simulink model "Navigation"  (R2021b)
settings: Solver=VariableStepAuto  StartTime=0.0  StopTime=10.0  RelTol=1e-3
settings Model: Creator=camil  LastModifiedBy=Paul

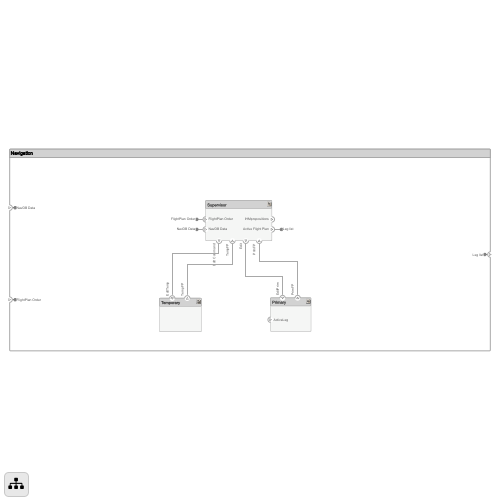
[thumbnail: Simulink's stored preview of the top-level diagram]
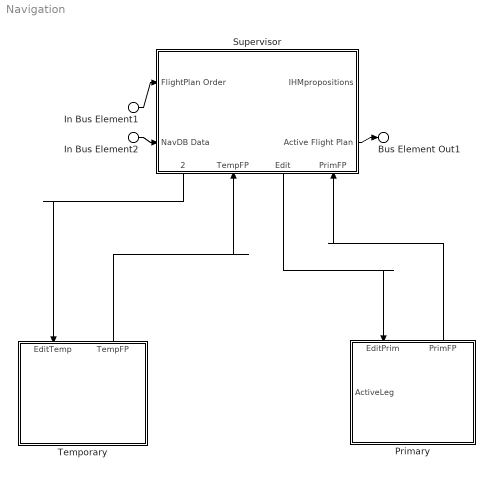
== system Navigation ==
  In Bus Element2 : Inport  PortName=NavDB Data
  In Bus Element1 : Inport  Port=2  PortName=FlightPlan Order
  Primary : Subsystem
      settings: PortSchema="{\"entries\":[{\"content\":{\"headerSize\":26,\"margin\":15,\"minimumSpacing\":25,\"sides\":[{\"content\":{\"connectorIds\":[\"In1\"]},\"type\":\"ConnectorPlacement.EquallySpacedRectSide\",\"uuid\":\"d7326126-d76c-444c-862a-2f0106f816d1\"},{\"content\":{\"connectorIds\":[],\"side\":\"RIGHT\"},\"type\":\"ConnectorPlacement.EquallySpacedRectSide\",\"uuid\":\"2601f9d1-3d71-4e08-9edb-3531e4b048a4\"},{\"content\":{\"connectorIds\":[\"In2\",\"Out1\"],\"side\":\"TOP\"},\"type\":\"ConnectorPlacement.EquallySpacedRectSide\",\"uuid\":\"741cf5f4-667e-43d2-9509-c9ba3ad46b0e\"}]},\"type\":\"ConnectorPlacement.EquallySpacedConnector\",\"uuid\":\"c4d920bd-28a0-4f0b-9ee2-ed60ff349b07\"}],\"packageUris\":[\"http://schema.mathworks.com/mf0/Connector/R2020b\"],\"version\":\"1.0\"}"
  Supervisor : Subsystem
      settings: PortSchema="{\"entries\":[{\"content\":{\"headerSize\":26,\"margin\":15,\"minimumSpacing\":25,\"sides\":[{\"content\":{\"connectorIds\":[\"In4\",\"In2\"]},\"type\":\"ConnectorPlacement.EquallySpacedRectSide\",\"uuid\":\"d7326126-d76c-444c-862a-2f0106f816d1\"},{\"content\":{\"connectorIds\":[\"Out1\",\"Out4\"],\"side\":\"RIGHT\"},\"type\":\"ConnectorPlacement.EquallySpacedRectSide\",\"uuid\":\"2601f9d1-3d71-4e08-9edb-3531e4b048a4\"},{\"content\":{\"connectorIds\":[],\"side\":\"TOP\"},\"type\":\"ConnectorPlacement.EquallySpacedRectSide\",\"uuid\":\"741cf5f4-667e-43d2-9509-c9ba3ad46b0e\"},{\"content\":{\"connectorIds\":[\"Out2\",\"In1\",\"Out3\",\"In3\"],\"side\":\"BOTTOM\"},\"type\":\"ConnectorPlacement.EquallySpacedRectSide\",\"uuid\":\"633d5e42-bd32-4027-bd9b-07f9504a1e08\"}]},\"type\":\"ConnectorPlacement.EquallySpacedConnector\",\"uuid\":\"c4d920bd-28a0-4f0b-9ee2-ed60ff349b07\"}],\"packageUris\":[\"http://schema.mathworks.com/mf0/Connector/R2020b\"],\"version\":\"1.0\"}"
  Temporary : Subsystem
      settings: PortSchema="{\"entries\":[{\"content\":{\"headerSize\":26,\"margin\":15,\"minimumSpacing\":25,\"sides\":[{\"content\":{\"connectorIds\":[]},\"type\":\"ConnectorPlacement.EquallySpacedRectSide\",\"uuid\":\"d7326126-d76c-444c-862a-2f0106f816d1\"},{\"content\":{\"connectorIds\":[],\"side\":\"RIGHT\"},\"type\":\"ConnectorPlacement.EquallySpacedRectSide\",\"uuid\":\"2601f9d1-3d71-4e08-9edb-3531e4b048a4\"},{\"content\":{\"connectorIds\":[\"In1\",\"Out1\"],\"side\":\"TOP\"},\"type\":\"ConnectorPlacement.EquallySpacedRectSide\",\"uuid\":\"741cf5f4-667e-43d2-9509-c9ba3ad46b0e\"}]},\"type\":\"ConnectorPlacement.EquallySpacedConnector\",\"uuid\":\"c4d920bd-28a0-4f0b-9ee2-ed60ff349b07\"}],\"packageUris\":[\"http://schema.mathworks.com/mf0/Connector/R2020b\"],\"version\":\"1.0\"}"
  Bus Element Out1 : Outport  RequirementInfo={} %GIDa_63419fd0_dcd8_4c60_9f87_9bda1864630e  PortName=Leg list
  wires:
  In Bus Element1/1 -> Supervisor/4(FlightPlan Order)
  Supervisor/4(Active Flight Plan) -> Bus Element Out1/1
  Supervisor/2(Edit Command) -> Temporary/1(EditTemp)
  Temporary/1(TempFP) -> Supervisor/1(TempFP)
  Supervisor/3(Edit) -> Primary/2(EditPrim)
  Primary/1(PrimFP) -> Supervisor/3(PrimFP)
  In Bus Element2/1 -> Supervisor/2(NavDB Data)

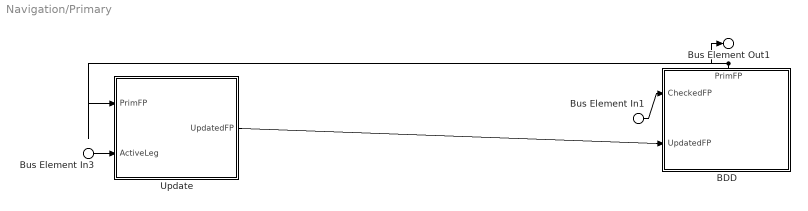
== system Navigation/Primary ==
  Bus Element In3 : Inport  PortName=ActiveLeg
  Bus Element In1 : Inport  Port=2  PortName=EditPrim
  BDD : Subsystem
      settings: PortSchema="{\"entries\":[{\"content\":{\"headerSize\":26,\"margin\":15,\"minimumSpacing\":25,\"sides\":[{\"content\":{\"connectorIds\":[\"In1\",\"In2\"]},\"type\":\"ConnectorPlacement.EquallySpacedRectSide\",\"uuid\":\"3f380961-0284-498f-9d20-a77cf1fdb000\"},{\"content\":{\"connectorIds\":[],\"side\":\"RIGHT\"},\"type\":\"ConnectorPlacement.EquallySpacedRectSide\",\"uuid\":\"c1cf40f6-b0eb-4111-9692-6c9c6cd53873\"},{\"content\":{\"connectorIds\":[\"Out1\"],\"side\":\"TOP\"},\"type\":\"ConnectorPlacement.EquallySpacedRectSide\",\"uuid\":\"4dc1c299-4e42-423b-9cac-e2e11c6bf6b6\"}]},\"type\":\"ConnectorPlacement.EquallySpacedConnector\",\"uuid\":\"af3a7563-dfec-45e0-bdfa-51dd28b27463\"}],\"packageUris\":[\"http://schema.mathworks.com/mf0/Connector/R2020b\"],\"version\":\"1.0\"}"
  Update : Subsystem
      settings: PortSchema="{\"entries\":[{\"content\":{\"headerSize\":26,\"margin\":15,\"minimumSpacing\":25,\"sides\":[{\"content\":{\"connectorIds\":[\"In1\",\"In2\"]},\"type\":\"ConnectorPlacement.EquallySpacedRectSide\",\"uuid\":\"3f380961-0284-498f-9d20-a77cf1fdb000\"},{\"content\":{\"connectorIds\":[\"Out1\"],\"side\":\"RIGHT\"},\"type\":\"ConnectorPlacement.EquallySpacedRectSide\",\"uuid\":\"c1cf40f6-b0eb-4111-9692-6c9c6cd53873\"},{\"content\":{\"connectorIds\":[],\"side\":\"TOP\"},\"type\":\"ConnectorPlacement.EquallySpacedRectSide\",\"uuid\":\"4dc1c299-4e42-423b-9cac-e2e11c6bf6b6\"}]},\"type\":\"ConnectorPlacement.EquallySpacedConnector\",\"uuid\":\"af3a7563-dfec-45e0-bdfa-51dd28b27463\"}],\"packageUris\":[\"http://schema.mathworks.com/mf0/Connector/R2020b\"],\"version\":\"1.0\"}"
  Bus Element Out1 : Outport  PortName=PrimFP
  wires:
  BDD/1(PrimFP) -> Update/1(PrimFP), Bus Element Out1/1
  Update/1(UpdatedFP) -> BDD/2(UpdatedFP)
  Bus Element In3/1 -> Update/2(ActiveLeg)
  Bus Element In1/1 -> BDD/1(CheckedFP)

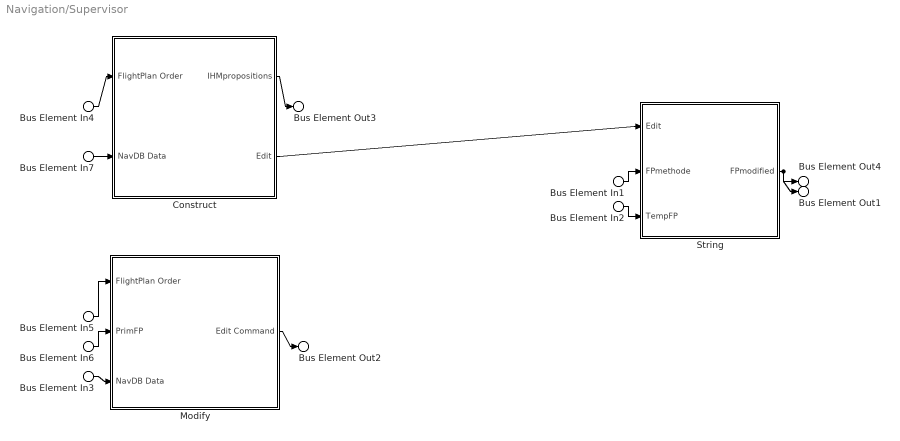
== system Navigation/Supervisor ==
  Bus Element In2 : Inport  PortName=TempFP
  Bus Element In3 : Inport  Port=2  PortName=NavDB Data
  Bus Element In7 : Inport  Port=2  PortName=NavDB Data
  Bus Element In6 : Inport  Port=3  PortName=PrimFP
  Bus Element In1 : Inport  Port=4  PortName=FlightPlan Order
  Bus Element In4 : Inport  Port=4  PortName=FlightPlan Order
  Bus Element In5 : Inport  Port=4  PortName=FlightPlan Order
  Construct : Subsystem
      settings: PortSchema="{\"entries\":[{\"content\":{\"headerSize\":26,\"margin\":15,\"minimumSpacing\":25,\"sides\":[{\"content\":{\"connectorIds\":[\"In1\",\"In2\"]},\"type\":\"ConnectorPlacement.EquallySpacedRectSide\",\"uuid\":\"4db80683-d003-4925-8eb8-5b8f8e0ba335\"},{\"content\":{\"connectorIds\":[\"Out1\",\"Out2\"],\"side\":\"RIGHT\"},\"type\":\"ConnectorPlacement.EquallySpacedRectSide\",\"uuid\":\"a8cdf0a8-cffb-416a-b4b0-3864e5651e68\"},{\"content\":{\"connectorIds\":[],\"side\":\"TOP\"},\"type\":\"ConnectorPlacement.EquallySpacedRectSide\",\"uuid\":\"9708d04f-d627-431e-b0fe-10b59962e11a\"}]},\"type\":\"ConnectorPlacement.EquallySpacedConnector\",\"uuid\":\"0a4dba50-ccc1-44d0-bfae-15615dd6a9d9\"}],\"packageUris\":[\"http://schema.mathworks.com/mf0/Connector/R2020b\"],\"version\":\"1.0\"}"
  Modify : Subsystem
      settings: PortSchema="{\"entries\":[{\"content\":{\"headerSize\":26,\"margin\":15,\"minimumSpacing\":25,\"sides\":[{\"content\":{\"connectorIds\":[\"In1\",\"In2\",\"In3\"]},\"type\":\"ConnectorPlacement.EquallySpacedRectSide\",\"uuid\":\"3f380961-0284-498f-9d20-a77cf1fdb000\"},{\"content\":{\"connectorIds\":[\"Out1\"],\"side\":\"RIGHT\"},\"type\":\"ConnectorPlacement.EquallySpacedRectSide\",\"uuid\":\"c1cf40f6-b0eb-4111-9692-6c9c6cd53873\"},{\"content\":{\"connectorIds\":[],\"side\":\"TOP\"},\"type\":\"ConnectorPlacement.EquallySpacedRectSide\",\"uuid\":\"4dc1c299-4e42-423b-9cac-e2e11c6bf6b6\"}]},\"type\":\"ConnectorPlacement.EquallySpacedConnector\",\"uuid\":\"af3a7563-dfec-45e0-bdfa-51dd28b27463\"}],\"packageUris\":[\"http://schema.mathworks.com/mf0/Connector/R2020b\"],\"version\":\"1.0\"}"
  String : Subsystem
      settings: PortSchema="{\"entries\":[{\"content\":{\"headerSize\":26,\"margin\":15,\"minimumSpacing\":25,\"sides\":[{\"content\":{\"connectorIds\":[\"In1\",\"In2\",\"In3\"]},\"type\":\"ConnectorPlacement.EquallySpacedRectSide\",\"uuid\":\"4db80683-d003-4925-8eb8-5b8f8e0ba335\"},{\"content\":{\"connectorIds\":[\"Out1\"],\"side\":\"RIGHT\"},\"type\":\"ConnectorPlacement.EquallySpacedRectSide\",\"uuid\":\"a8cdf0a8-cffb-416a-b4b0-3864e5651e68\"},{\"content\":{\"connectorIds\":[],\"side\":\"TOP\"},\"type\":\"ConnectorPlacement.EquallySpacedRectSide\",\"uuid\":\"9708d04f-d627-431e-b0fe-10b59962e11a\"}]},\"type\":\"ConnectorPlacement.EquallySpacedConnector\",\"uuid\":\"0a4dba50-ccc1-44d0-bfae-15615dd6a9d9\"}],\"packageUris\":[\"http://schema.mathworks.com/mf0/Connector/R2020b\"],\"version\":\"1.0\"}"
  Bus Element Out3 : Outport  PortName=IHMpropositions
  Bus Element Out2 : Outport  Port=2  PortName=Edit Command
  Bus Element Out4 : Outport  Port=3  PortName=Edit
  Bus Element Out1 : Outport  Port=4  PortName=Active Flight Plan
  wires:
  Bus Element In1/1 -> String/2(FPmethode)
  Bus Element In4/1 -> Construct/1(FlightPlan Order)
  Bus Element In5/1 -> Modify/1(FlightPlan Order)
  Bus Element In6/1 -> Modify/2(PrimFP)
  Modify/1(Edit Command) -> Bus Element Out2/1
  Construct/2(Edit) -> String/1(Edit)
  Bus Element In2/1 -> String/3(TempFP)
  String/1(FPmodified) -> Bus Element Out4/1, Bus Element Out1/1
  Construct/1(IHMpropositions) -> Bus Element Out3/1
  Bus Element In3/1 -> Modify/3(NavDB Data)
  Bus Element In7/1 -> Construct/2(NavDB Data)

== system Navigation/Temporary ==
  Bus Element In1 : Inport  PortName=EditTemp
  Bus Element Out1 : Outport  PortName=TempFP

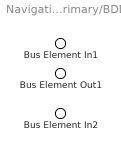
== system Navigation/Primary/BDD ==
  Bus Element In1 : Inport  PortName=CheckedFP
  Bus Element In2 : Inport  Port=2  PortName=UpdatedFP
  Bus Element Out1 : Outport  PortName=PrimFP

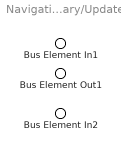
== system Navigation/Primary/Update ==
  Bus Element In1 : Inport  PortName=PrimFP
  Bus Element In2 : Inport  Port=2  PortName=ActiveLeg
  Bus Element Out1 : Outport  PortName=UpdatedFP

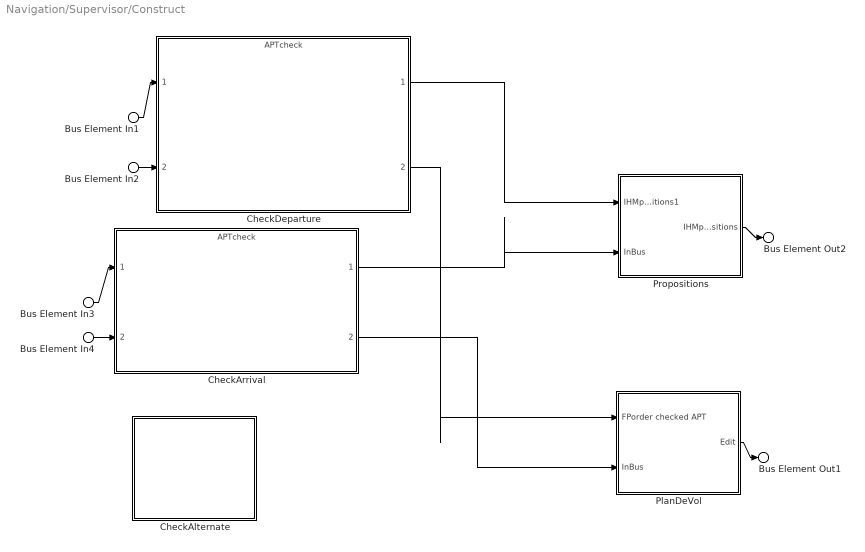
== system Navigation/Supervisor/Construct ==
  Bus Element In1 : Inport  PortName=FlightPlan Order
  Bus Element In3 : Inport  PortName=FlightPlan Order
  Bus Element In2 : Inport  Port=2  PortName=NavDB Data
  Bus Element In4 : Inport  Port=2  PortName=NavDB Data
  CheckAlternate : Subsystem
      settings: PortSchema="{\"entries\":[{\"content\":{\"headerSize\":26,\"margin\":15,\"minimumSpacing\":25,\"sides\":[{\"content\":{\"connectorIds\":[]},\"type\":\"ConnectorPlacement.EquallySpacedRectSide\",\"uuid\":\"3f380961-0284-498f-9d20-a77cf1fdb000\"},{\"content\":{\"connectorIds\":[],\"side\":\"RIGHT\"},\"type\":\"ConnectorPlacement.EquallySpacedRectSide\",\"uuid\":\"c1cf40f6-b0eb-4111-9692-6c9c6cd53873\"},{\"content\":{\"connectorIds\":[],\"side\":\"TOP\"},\"type\":\"ConnectorPlacement.EquallySpacedRectSide\",\"uuid\":\"4dc1c299-4e42-423b-9cac-e2e11c6bf6b6\"}]},\"type\":\"ConnectorPlacement.EquallySpacedConnector\",\"uuid\":\"af3a7563-dfec-45e0-bdfa-51dd28b27463\"}],\"packageUris\":[\"http://schema.mathworks.com/mf0/Connector/R2020b\"],\"version\":\"1.0\"}"
  CheckArrival : ModelReference  ModelNameDialog=APTcheck  SimulationMode=Normal  ModelReferenceVersion=1.1
      settings: PortSchema="{\"entries\":[{\"content\":{\"headerSize\":38,\"margin\":15,\"minimumSpacing\":25,\"sides\":[{\"content\":{\"connectorIds\":[\"In1\",\"In2\"]},\"type\":\"ConnectorPlacement.EquallySpacedRectSide\",\"uuid\":\"3f380961-0284-498f-9d20-a77cf1fdb000\"},{\"content\":{\"connectorIds\":[\"Out1\",\"Out2\"],\"side\":\"RIGHT\"},\"type\":\"ConnectorPlacement.EquallySpacedRectSide\",\"uuid\":\"c1cf40f6-b0eb-4111-9692-6c9c6cd53873\"},{\"content\":{\"connectorIds\":[],\"side\":\"TOP\"},\"type\":\"ConnectorPlacement.EquallySpacedRectSide\",\"uuid\":\"4dc1c299-4e42-423b-9cac-e2e11c6bf6b6\"}]},\"type\":\"ConnectorPlacement.EquallySpacedConnector\",\"uuid\":\"af3a7563-dfec-45e0-bdfa-51dd28b27463\"}],\"packageUris\":[\"http://schema.mathworks.com/mf0/Connector/R2020b\"],\"version\":\"1.0\"}"
  CheckDeparture : ModelReference  ModelNameDialog=APTcheck  SimulationMode=Normal  ModelReferenceVersion=1.1
      settings: PortSchema="{\"entries\":[{\"content\":{\"headerSize\":38,\"margin\":15,\"minimumSpacing\":25,\"sides\":[{\"content\":{\"connectorIds\":[\"In1\",\"In2\"]},\"type\":\"ConnectorPlacement.EquallySpacedRectSide\",\"uuid\":\"3f380961-0284-498f-9d20-a77cf1fdb000\"},{\"content\":{\"connectorIds\":[\"Out1\",\"Out2\"],\"side\":\"RIGHT\"},\"type\":\"ConnectorPlacement.EquallySpacedRectSide\",\"uuid\":\"c1cf40f6-b0eb-4111-9692-6c9c6cd53873\"},{\"content\":{\"connectorIds\":[],\"side\":\"TOP\"},\"type\":\"ConnectorPlacement.EquallySpacedRectSide\",\"uuid\":\"4dc1c299-4e42-423b-9cac-e2e11c6bf6b6\"}]},\"type\":\"ConnectorPlacement.EquallySpacedConnector\",\"uuid\":\"af3a7563-dfec-45e0-bdfa-51dd28b27463\"}],\"packageUris\":[\"http://schema.mathworks.com/mf0/Connector/R2020b\"],\"version\":\"1.0\"}"
  PlanDeVol : Subsystem
      settings: PortSchema="{\"entries\":[{\"content\":{\"headerSize\":26,\"margin\":15,\"minimumSpacing\":25,\"sides\":[{\"content\":{\"connectorIds\":[\"In1\",\"In2\"]},\"type\":\"ConnectorPlacement.EquallySpacedRectSide\",\"uuid\":\"3f380961-0284-498f-9d20-a77cf1fdb000\"},{\"content\":{\"connectorIds\":[\"Out1\"],\"side\":\"RIGHT\"},\"type\":\"ConnectorPlacement.EquallySpacedRectSide\",\"uuid\":\"c1cf40f6-b0eb-4111-9692-6c9c6cd53873\"},{\"content\":{\"connectorIds\":[],\"side\":\"TOP\"},\"type\":\"ConnectorPlacement.EquallySpacedRectSide\",\"uuid\":\"4dc1c299-4e42-423b-9cac-e2e11c6bf6b6\"}]},\"type\":\"ConnectorPlacement.EquallySpacedConnector\",\"uuid\":\"af3a7563-dfec-45e0-bdfa-51dd28b27463\"}],\"packageUris\":[\"http://schema.mathworks.com/mf0/Connector/R2020b\"],\"version\":\"1.0\"}"
  Propositions : Subsystem
      settings: PortSchema="{\"entries\":[{\"content\":{\"headerSize\":26,\"margin\":15,\"minimumSpacing\":25,\"sides\":[{\"content\":{\"connectorIds\":[\"In1\",\"In2\"]},\"type\":\"ConnectorPlacement.EquallySpacedRectSide\",\"uuid\":\"3f380961-0284-498f-9d20-a77cf1fdb000\"},{\"content\":{\"connectorIds\":[\"Out1\"],\"side\":\"RIGHT\"},\"type\":\"ConnectorPlacement.EquallySpacedRectSide\",\"uuid\":\"c1cf40f6-b0eb-4111-9692-6c9c6cd53873\"},{\"content\":{\"connectorIds\":[],\"side\":\"TOP\"},\"type\":\"ConnectorPlacement.EquallySpacedRectSide\",\"uuid\":\"4dc1c299-4e42-423b-9cac-e2e11c6bf6b6\"}]},\"type\":\"ConnectorPlacement.EquallySpacedConnector\",\"uuid\":\"af3a7563-dfec-45e0-bdfa-51dd28b27463\"}],\"packageUris\":[\"http://schema.mathworks.com/mf0/Connector/R2020b\"],\"version\":\"1.0\"}"
  Bus Element Out2 : Outport  PortName=IHMpropositions
  Bus Element Out1 : Outport  Port=2  PortName=Edit
  wires:
  CheckDeparture/1 -> Propositions/1(IHMpropositions1)
  CheckArrival/1 -> Propositions/2(InBus)
  Propositions/1(IHMpropositions) -> Bus Element Out2/1
  CheckDeparture/2 -> PlanDeVol/1(FPorder checked APT)
  CheckArrival/2 -> PlanDeVol/2(InBus)
  PlanDeVol/1(Edit) -> Bus Element Out1/1
  Bus Element In1/1 -> CheckDeparture/1
  Bus Element In3/1 -> CheckArrival/1
  Bus Element In2/1 -> CheckDeparture/2
  Bus Element In4/1 -> CheckArrival/2

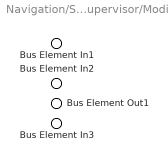
== system Navigation/Supervisor/Modify ==
  Bus Element In1 : Inport  PortName=FlightPlan Order
  Bus Element In2 : Inport  Port=2  PortName=PrimFP
  Bus Element In3 : Inport  Port=3  PortName=NavDB Data
  Bus Element Out1 : Outport  PortName=Edit Command

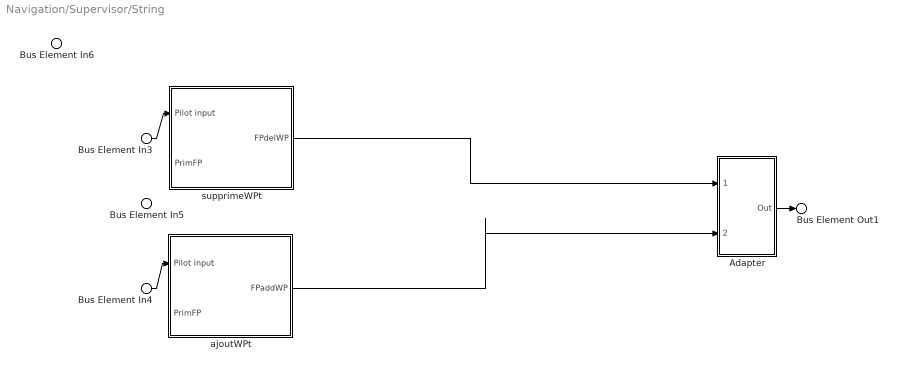
== system Navigation/Supervisor/String ==
  Bus Element In6 : Inport  PortName=Edit
  Bus Element In3 : Inport  Port=2  PortName=FPmethode
  Bus Element In4 : Inport  Port=2  PortName=FPmethode
  Bus Element In5 : Inport  Port=3  PortName=TempFP
  Adapter : Subsystem
      settings: PortSchema="{\"entries\":[{\"content\":{\"margin\":10,\"minimumSpacing\":15,\"sides\":[{\"content\":{\"connectorIds\":[\"In1\",\"In2\"]},\"type\":\"ConnectorPlacement.EquallySpacedRectSide\",\"uuid\":\"4db80683-d003-4925-8eb8-5b8f8e0ba335\"},{\"content\":{\"connectorIds\":[\"Out1\"],\"side\":\"RIGHT\"},\"type\":\"ConnectorPlacement.EquallySpacedRectSide\",\"uuid\":\"a8cdf0a8-cffb-416a-b4b0-3864e5651e68\"},{\"content\":{\"connectorIds\":[],\"side\":\"TOP\"},\"type\":\"ConnectorPlacement.EquallySpacedRectSide\",\"uuid\":\"9708d04f-d627-431e-b0fe-10b59962e11a\"}]},\"type\":\"ConnectorPlacement.EquallySpacedConnector\",\"uuid\":\"0a4dba50-ccc1-44d0-bfae-15615dd6a9d9\"}],\"packageUris\":[\"http://schema.mathworks.com/mf0/Connector/R2020b\"],\"version\":\"1.0\"}"
  ajoutWPt : Subsystem
      settings: PortSchema="{\"entries\":[{\"content\":{\"headerSize\":26,\"margin\":15,\"minimumSpacing\":25,\"sides\":[{\"content\":{\"connectorIds\":[\"In1\",\"In2\"]},\"type\":\"ConnectorPlacement.EquallySpacedRectSide\",\"uuid\":\"4db80683-d003-4925-8eb8-5b8f8e0ba335\"},{\"content\":{\"connectorIds\":[\"Out1\"],\"side\":\"RIGHT\"},\"type\":\"ConnectorPlacement.EquallySpacedRectSide\",\"uuid\":\"a8cdf0a8-cffb-416a-b4b0-3864e5651e68\"},{\"content\":{\"connectorIds\":[],\"side\":\"TOP\"},\"type\":\"ConnectorPlacement.EquallySpacedRectSide\",\"uuid\":\"9708d04f-d627-431e-b0fe-10b59962e11a\"}]},\"type\":\"ConnectorPlacement.EquallySpacedConnector\",\"uuid\":\"0a4dba50-ccc1-44d0-bfae-15615dd6a9d9\"}],\"packageUris\":[\"http://schema.mathworks.com/mf0/Connector/R2020b\"],\"version\":\"1.0\"}"
  supprimeWPt : Subsystem
      settings: PortSchema="{\"entries\":[{\"content\":{\"headerSize\":26,\"margin\":15,\"minimumSpacing\":25,\"sides\":[{\"content\":{\"connectorIds\":[\"In1\",\"In2\"]},\"type\":\"ConnectorPlacement.EquallySpacedRectSide\",\"uuid\":\"4db80683-d003-4925-8eb8-5b8f8e0ba335\"},{\"content\":{\"connectorIds\":[\"Out1\"],\"side\":\"RIGHT\"},\"type\":\"ConnectorPlacement.EquallySpacedRectSide\",\"uuid\":\"a8cdf0a8-cffb-416a-b4b0-3864e5651e68\"},{\"content\":{\"connectorIds\":[],\"side\":\"TOP\"},\"type\":\"ConnectorPlacement.EquallySpacedRectSide\",\"uuid\":\"9708d04f-d627-431e-b0fe-10b59962e11a\"}]},\"type\":\"ConnectorPlacement.EquallySpacedConnector\",\"uuid\":\"0a4dba50-ccc1-44d0-bfae-15615dd6a9d9\"}],\"packageUris\":[\"http://schema.mathworks.com/mf0/Connector/R2020b\"],\"version\":\"1.0\"}"
  Bus Element Out1 : Outport  PortName=FPmodified
  wires:
  ? -> ajoutWPt/2(PrimFP)
  ? -> supprimeWPt/2(PrimFP)
  Bus Element In3/1 -> supprimeWPt/1(Pilot input)
  Bus Element In4/1 -> ajoutWPt/1(Pilot input)
  Adapter/1(Out) -> Bus Element Out1/1
  ajoutWPt/1(FPaddWP) -> Adapter/2(FPaddWP)
  supprimeWPt/1(FPdelWP) -> Adapter/1(FPmodified)

== system Navigation/Supervisor/Construct/CheckAlternate ==

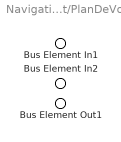
== system Navigation/Supervisor/Construct/PlanDeVol ==
  Bus Element In1 : Inport  PortName=FPorder checked APT
  Bus Element In2 : Inport  Port=2  PortName=InBus
  Bus Element Out1 : Outport  PortName=Edit

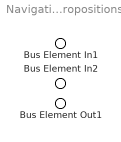
== system Navigation/Supervisor/Construct/Propositions ==
  Bus Element In1 : Inport  PortName=IHMpropositions1
  Bus Element In2 : Inport  Port=2  PortName=InBus
  Bus Element Out1 : Outport  PortName=IHMpropositions

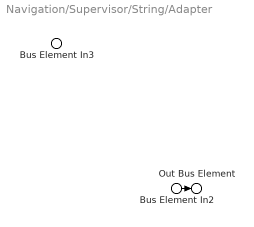
== system Navigation/Supervisor/String/Adapter ==
  Bus Element In3 : Inport  PortName=FPmodified
  Bus Element In2 : Inport  Port=2  PortName=FPaddWP
  Out Bus Element : Outport  PortName=Out
  wires:
  Bus Element In2/1 -> Out Bus Element/1

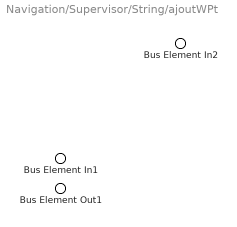
== system Navigation/Supervisor/String/ajoutWPt ==
  Bus Element In2 : Inport  PortName=Pilot input
  Bus Element In1 : Inport  Port=2  PortName=PrimFP
  Bus Element Out1 : Outport  PortName=FPaddWP

== system Navigation/Supervisor/String/supprimeWPt ==
  Bus Element In2 : Inport  PortName=Pilot input
  Bus Element In1 : Inport  Port=2  PortName=PrimFP
  Bus Element Out1 : Outport  PortName=FPdelWP
